simulink model "EEG_Characterization_Model"  (R2024b)
settings: Solver=VariableStepAuto  StartTime=0.0  StopTime=1  RelTol=1e-3  AbsTol=1e-3
libraries: fl_lib x28, nesl_utility x7
settings Model: Creator=RyanCorp  LastModifiedBy=RyanCorp
settings SolverCC: AutoScaleAbsTol=off  AlgebraicLoopSolver=TrustRegion  MaxZcPerStep=1
settings DebuggingCC: UnconnectedInputMsg=warning  UnconnectedOutputMsg=warning  UnconnectedLineMsg=warning  SymbolicDimsDataTypeCodeGenerationDiagnostic=none
settings ModelReferenceCC: EnableRefExpFcnMdlSchedulingChecks=on
settings SFSimCC: CustomCodeUndefinedFunction=UseInterfaceOnly
settings RTWCC: GPUComputeCapability=3.5  DLArmComputeVersion=19.05
settings SimscapeCC: SimscapeLogType=all  SimscapeLogSimulationStatistics=on  SimscapeLogDataHistory=10000

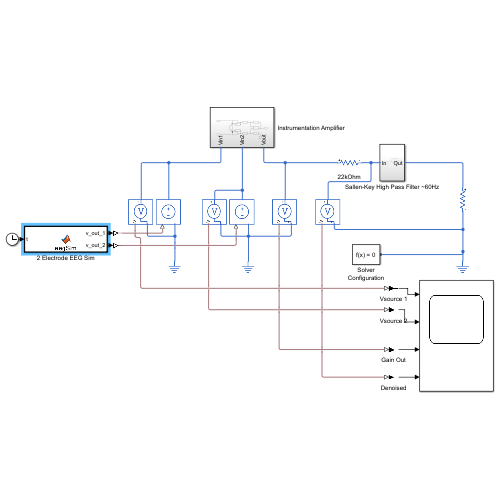
[thumbnail: Simulink's stored preview of the top-level diagram]
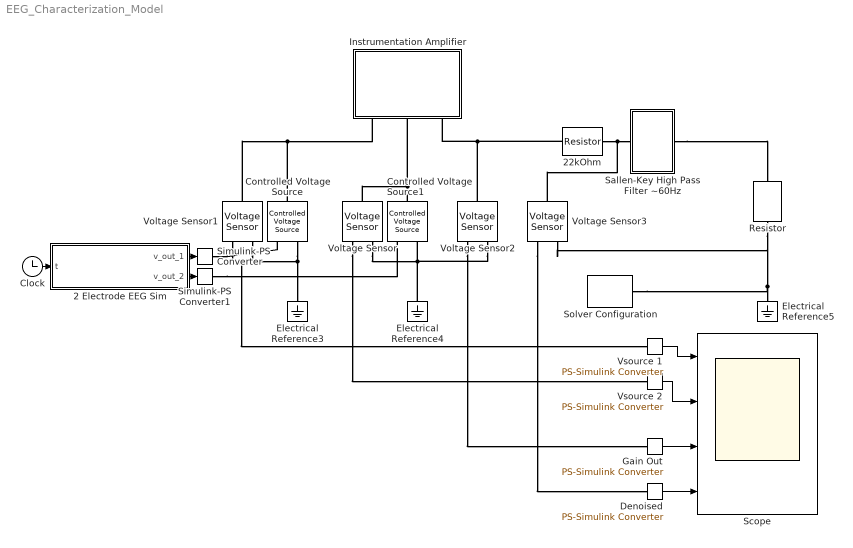
== system EEG_Characterization_Model ==
  2 Electrode EEG Sim : MATLAB Function  TreatAsAtomicUnit=on  SystemSampleTime=0.001
  22kOhm : fl_lib/Electrical/Electrical Elements/Resistor  R=22 kOhm  i_specify=off  i_priority=None  i=0 A  i_nominal_specify=off  i_nominal_value=1  i_nominal_unit=A  v_specify=off  v_priority=None  v=0 V  v_nominal_specify=off  v_nominal_value=1  v_nominal_unit=V
  Clock : Clock
  Controlled Voltage Source : fl_lib/Electrical/Electrical Sources/Controlled Voltage Source
  Controlled Voltage Source1 : fl_lib/Electrical/Electrical Sources/Controlled Voltage Source
  Denoised : nesl_utility/PS-Simulink Converter  PhysicalDomain=network_engine_domain  SubClassName=ps_output  LeftPortType=input  RightPortType=output  PseudoPeriodic=off  Frequencies=[]  VectorFormat=inherit  Unit=inherit  AffineConversion=off
  Electrical Reference3 : fl_lib/Electrical/Electrical Elements/Electrical Reference
  Electrical Reference4 : fl_lib/Electrical/Electrical Elements/Electrical Reference
  Electrical Reference5 : fl_lib/Electrical/Electrical Elements/Electrical Reference
  Gain Out : nesl_utility/PS-Simulink Converter  PhysicalDomain=network_engine_domain  SubClassName=ps_output  LeftPortType=input  RightPortType=output  PseudoPeriodic=off  Frequencies=[]  VectorFormat=inherit  Unit=inherit  AffineConversion=off
  Instrumentation Amplifier : Subsystem
  Resistor : fl_lib/Electrical/Electrical Elements/Resistor  R=32 Ohm  i_specify=off  i_priority=None  i=0 A  i_nominal_specify=off  i_nominal_value=1  i_nominal_unit=A  v_specify=off  v_priority=None  v=0 V  v_nominal_specify=off  v_nominal_value=1  v_nominal_unit=V
  Sallen-Key High Pass Filter ~60Hz : Subsystem
  Scope : Scope  NumInputPorts=4
  Simulink-PS Converter : nesl_utility/Simulink-PS Converter  PhysicalDomain=network_engine_domain  SubClassName=ps_input  LeftPortType=input  RightPortType=output  PseudoPeriodic=off  Frequencies=[]  NoiseDistribution=none  NoiseParameters=[]  Unit=1  AffineConversion=off  FilteringAndDerivatives=provide  SimscapeFilterOrder=1  InputFilterTimeConstant=0.001  UdotUserProvided=0
  Simulink-PS Converter1 : nesl_utility/Simulink-PS Converter  PhysicalDomain=network_engine_domain  SubClassName=ps_input  LeftPortType=input  RightPortType=output  PseudoPeriodic=off  Frequencies=[]  NoiseDistribution=none  NoiseParameters=[]  Unit=1  AffineConversion=off  FilteringAndDerivatives=provide  SimscapeFilterOrder=1  InputFilterTimeConstant=0.001  UdotUserProvided=0
  Solver Configuration : nesl_utility/Solver Configuration  PhysicalDomain=network_engine_domain  SubClassName=solver  LeftPortType=input  RightPortType=generic  Tones=[]  Harmonics=[]  SimulateNoise=off  Profile=off  UseLocalSampling=off  EnableSwitchedLinearOptims=on  FrequencyDomain=off  UseCCode=off  RelTol=0.001  AbsTol=1e-06  MinStep=1e-09  ToWorkspace=off  RevertToSquareIcSolve=off  NumHomotopyIterations=100  PhasorMode=off  PhasorModeNumHarmonics=1  ConsistencySolver=NEWTON_XTOL_AFTER_FTOL  IndexReductionMethod=DerivativeReplacement  DoDC=off  ResidualTolerance=1e-09  ConsistencyTolSource=GLOBAL  ConsistencyAbsTol=0.001  ConsistencyRelTol=0.001  ConsistencyTolFactor=0.001  UseLocalSolver=off  LocalSolverChoice=NE_BACKWARD_EULER_ADVANCER  ResolveIndetEquations=on  FunctionEvalNumThread=1  LocalSolverSampleTime=0.001  DoFixedCost=off  MaxNonlinIter=3  MaxModeIter=2  ComputeImpulses=off  ImpulseIterations=2  LinearAlgebra=auto  LinearAlgebraNumThread=0  EquationFormulation=NE_TIME_EF  DelaysMemoryBudget=1024  AutomaticFiltering=on  FilteringTimeConstant=0.001  PartitionStorageMethod=AS_NEEDED  PartitionMemoryBudget=1024  PartitionMethod=ROBUST  MultibodyUseLocalSolver=off  MultibodyLocalSolverChoice=ODE1  MultibodyLocalSolverSampleTime=0.001
  Voltage Sensor{,1..3} (4 alike) : fl_lib/Electrical/Electrical Sensors/Voltage Sensor
  Vsource 1 : nesl_utility/PS-Simulink Converter  PhysicalDomain=network_engine_domain  SubClassName=ps_output  LeftPortType=input  RightPortType=output  PseudoPeriodic=off  Frequencies=[]  VectorFormat=inherit  Unit=inherit  AffineConversion=off
  Vsource 2 : nesl_utility/PS-Simulink Converter  PhysicalDomain=network_engine_domain  SubClassName=ps_output  LeftPortType=input  RightPortType=output  PseudoPeriodic=off  Frequencies=[]  VectorFormat=inherit  Unit=inherit  AffineConversion=off
  wires:
  Vsource 1/1 -> Scope/1
  Vsource 2/1 -> Scope/2
  Clock/1 -> 2 Electrode EEG Sim/1(t)
  2 Electrode EEG Sim/1(v_out_1) -> Simulink-PS Converter/1
  2 Electrode EEG Sim/2(v_out_2) -> Simulink-PS Converter1/1
  Gain Out/1 -> Scope/3
  Denoised/1 -> Scope/4
  connections:
  Controlled Voltage Source/LConn1 -- Voltage Sensor1/LConn1 -- Instrumentation Amplifier/LConn1
  Voltage Sensor1/RConn1 -- Vsource 1/LConn1
  Voltage Sensor/RConn1 -- Vsource 2/LConn1
  Controlled Voltage Source1/LConn1 -- Voltage Sensor/LConn1 -- Instrumentation Amplifier/LConn2
  Simulink-PS Converter/RConn1 -- Controlled Voltage Source/RConn1
  Simulink-PS Converter1/RConn1 -- Controlled Voltage Source1/RConn1
  22kOhm/LConn1 -- Voltage Sensor2/LConn1 -- Instrumentation Amplifier/LConn3
  Voltage Sensor3/RConn1 -- Denoised/LConn1
  22kOhm/RConn1 -- Voltage Sensor3/LConn1 -- Sallen-Key High Pass Filter ~60Hz/LConn1
  Electrical Reference4/LConn1 -- Voltage Sensor2/RConn2 -- Voltage Sensor/RConn2 -- Controlled Voltage Source1/RConn2
  Controlled Voltage Source/RConn2 -- Voltage Sensor1/RConn2 -- Electrical Reference3/LConn1
  Solver Configuration/RConn1 -- Voltage Sensor3/RConn2 -- Resistor/RConn1 -- Electrical Reference5/LConn1
  Sallen-Key High Pass Filter ~60Hz/RConn1 -- Resistor/LConn1
  Voltage Sensor2/RConn1 -- Gain Out/LConn1

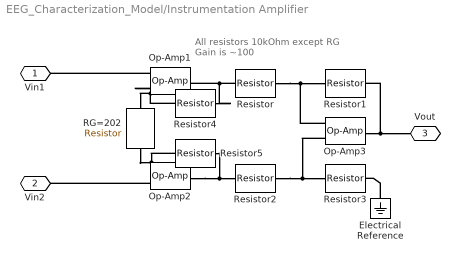
== system EEG_Characterization_Model/Instrumentation Amplifier ==
  note: All resistors 10kOhm except RG
      | Gain is ~100
  Electrical Reference : fl_lib/Electrical/Electrical Elements/Electrical Reference
  Op-Amp1 : fl_lib/Electrical/Electrical Elements/Op-Amp  outI_specify=off  outI_priority=None  outI=0 A  outI_nominal_specify=off  outI_nominal_value=1  outI_nominal_unit=A
  Op-Amp2 : fl_lib/Electrical/Electrical Elements/Op-Amp  outI_specify=off  outI_priority=None  outI=0 A  outI_nominal_specify=off  outI_nominal_value=1  outI_nominal_unit=A
  Op-Amp3 : fl_lib/Electrical/Electrical Elements/Op-Amp  outI_specify=off  outI_priority=None  outI=0 A  outI_nominal_specify=off  outI_nominal_value=1  outI_nominal_unit=A
  RG=202 : fl_lib/Electrical/Electrical Elements/Resistor  R=202 Ohm  i_specify=off  i_priority=None  i=0 A  i_nominal_specify=off  i_nominal_value=1  i_nominal_unit=A  v_specify=off  v_priority=None  v=0 V  v_nominal_specify=off  v_nominal_value=1  v_nominal_unit=V
  Resistor{,1..5} (6 alike) : fl_lib/Electrical/Electrical Elements/Resistor  R=10 kOhm  i_specify=off  i_priority=None  i=0 A  i_nominal_specify=off  i_nominal_value=1  i_nominal_unit=A  v_specify=off  v_priority=None  v=0 V  v_nominal_specify=off  v_nominal_value=1  v_nominal_unit=V
  Vin1 : PMIOPort  Side=Left
  Vin2 : PMIOPort  Port=2  Side=Left
  Vout : PMIOPort  Port=3  Side=Left
  connections:
  Op-Amp1/LConn1 -- Vin1/RConn1
  Resistor2/RConn1 -- Op-Amp3/LConn1 -- Resistor3/LConn1
  Resistor/LConn1 -- Resistor4/RConn1 -- Op-Amp1/RConn1
  Resistor/RConn1 -- Op-Amp3/LConn2 -- Resistor1/LConn1
  Op-Amp3/RConn1 -- Resistor1/RConn1 -- Vout/RConn1
  Op-Amp2/RConn1 -- Resistor5/RConn1 -- Resistor2/LConn1
  Op-Amp1/LConn2 -- Resistor4/LConn1 -- RG=202/LConn1
  Electrical Reference/LConn1 -- Resistor3/RConn1
  Resistor5/LConn1 -- RG=202/RConn1 -- Op-Amp2/LConn2
  Op-Amp2/LConn1 -- Vin2/RConn1

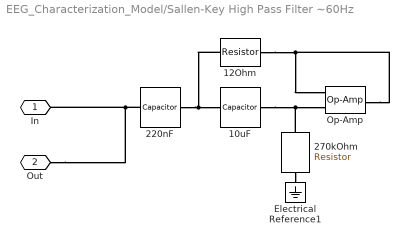
== system EEG_Characterization_Model/Sallen-Key High Pass Filter ~60Hz ==
  10uF : fl_lib/Electrical/Electrical Elements/Capacitor  c=10 uF  r=1e-6 Ohm  g=0 1/Ohm  i_specify=off  i_priority=None  i=0 A  i_nominal_specify=off  i_nominal_value=1  i_nominal_unit=A  v_specify=on  v_priority=None  v=0 V  v_nominal_specify=off  v_nominal_value=1  v_nominal_unit=V  vc_specify=off  vc_priority=High  vc=0 V  vc_nominal_specify=off  vc_nominal_value=1  vc_nominal_unit=V
  12Ohm : fl_lib/Electrical/Electrical Elements/Resistor  R=12 Ohm  i_specify=off  i_priority=None  i=0 A  i_nominal_specify=off  i_nominal_value=1  i_nominal_unit=A  v_specify=off  v_priority=None  v=0 V  v_nominal_specify=off  v_nominal_value=1  v_nominal_unit=V
  220nF : fl_lib/Electrical/Electrical Elements/Capacitor  c=220 nF  r=1e-6 Ohm  g=0 1/Ohm  i_specify=off  i_priority=None  i=0 A  i_nominal_specify=off  i_nominal_value=1  i_nominal_unit=A  v_specify=on  v_priority=None  v=0 V  v_nominal_specify=off  v_nominal_value=1  v_nominal_unit=V  vc_specify=off  vc_priority=High  vc=0 V  vc_nominal_specify=off  vc_nominal_value=1  vc_nominal_unit=V
  270kOhm : fl_lib/Electrical/Electrical Elements/Resistor  R=270 kOhm  i_specify=off  i_priority=None  i=0 A  i_nominal_specify=off  i_nominal_value=1  i_nominal_unit=A  v_specify=off  v_priority=None  v=0 V  v_nominal_specify=off  v_nominal_value=1  v_nominal_unit=V
  Electrical Reference1 : fl_lib/Electrical/Electrical Elements/Electrical Reference
  Op-Amp : fl_lib/Electrical/Electrical Elements/Op-Amp  outI_specify=off  outI_priority=None  outI=0 A  outI_nominal_specify=off  outI_nominal_value=1  outI_nominal_unit=A
  In : PMIOPort  Side=Left
  Out : PMIOPort  Port=2  Side=Right
  connections:
  10uF/RConn1 -- 270kOhm/LConn1 -- Op-Amp/LConn1
  220nF/RConn1 -- 12Ohm/RConn1 -- 10uF/LConn1
  Op-Amp/RConn1 -- 12Ohm/LConn1 -- Op-Amp/LConn2
  270kOhm/RConn1 -- Electrical Reference1/LConn1
  220nF/LConn1 -- Out/RConn1 -- In/RConn1

== matlab function EEG_Characterization_Model/2 Electrode EEG Sim ==
  data: t input; v_out_1 output; v_out_2 output
function [v_out_1, v_out_2] = eegSim(t)
% Simulates voltages from two EEG electrodes with added noise and outputs their differential

% DC offset voltage
dc_offset = 0.1;

% Electrode signal parameters (in microvolts)
amp1 = 50e-6;       % Amplitude for electrode 1
amp2 = 45e-6;       % Amplitude for electrode 2
freq1 = 10;         % Frequency in Hz (e.g., alpha wave)
freq2 = 10.5;       % Slight variation to simulate interference
phase2 = pi/6;      % Phase offset for second electrode

% Baseline DC drift (movement artifact/slow potential)
dc_drift = 10e-6 * sin(0.5 * 2 * pi * t);

% 60 Hz noise (simulate power line interference)
amp_60Hz = 5e-6;  % Adjust to fit realistic power line artifact amplitude
noise_60Hz = amp_60Hz * sin(2 * pi * 60 * t);

% General white noise
amp_white = 2e-6; % Standard deviation for Gaussian noise
white_noise1 = amp_white * randn();
white_noise2 = amp_white * randn();

% Final EEG electrode signals
v_out_1 = amp1 * sin(2 * pi * freq1 * t) + dc_drift + dc_offset + noise_60Hz + white_noise1;
v_out_2 = amp2 * sin(2 * pi * freq2 * t + phase2) + dc_offset + noise_60Hz + white_noise2;
